simulink model "Ejercicio2"  (R2018b)
settings: Solver=FixedStepAuto  StartTime=0.0  StopTime=100.0  FixedStep=0.01  RelTol=1e-3
undefined symbols (not defined in the file or in its folder): DiscIntNeverNeededParam
libraries: simulink x1
settings Model: EnablePacing=on  PacingRate=10  Creator=Edu  LastModifiedBy=Edu

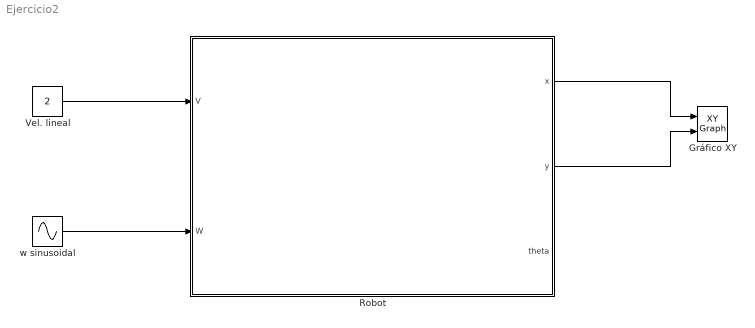
== system Ejercicio2 ==
  Gráfico XY : simulink/Sinks/XY Graph  xmin=-4  xmax=14  ymin=-4  ymax=14  st=-1
  Robot : Subsystem
  Vel. lineal : Constant  Value=2
  w sinusoidal : Sin  Amplitude=10  Frequency=10  SampleTime=0
  wires:
  Vel. lineal/1 -> Robot/1(V)
  Robot/1(x) -> Gráfico XY/1
  Robot/2(y) -> Gráfico XY/2
  w sinusoidal/1 -> Robot/2(W)

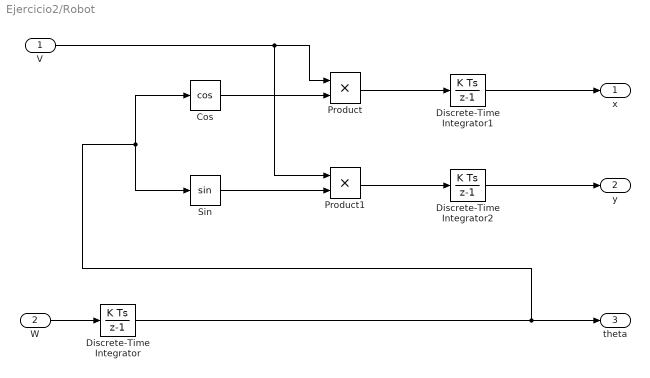
== system Ejercicio2/Robot ==
  V : Inport
  W : Inport  Port=2
  Cos : Trigonometry  Operator=cos
  Discrete-Time Integrator : DiscreteIntegrator  SampleTime=-1  ICPrevOutput=DiscIntNeverNeededParam  ICPrevScaledInput=DiscIntNeverNeededParam
  Discrete-Time Integrator1 : DiscreteIntegrator  InitialCondition=-4  SampleTime=-1  ICPrevOutput=DiscIntNeverNeededParam  ICPrevScaledInput=DiscIntNeverNeededParam
  Discrete-Time Integrator2 : DiscreteIntegrator  InitialCondition=-4  SampleTime=-1  ICPrevOutput=DiscIntNeverNeededParam  ICPrevScaledInput=DiscIntNeverNeededParam
  Product : Product
  Product1 : Product
  Sin : Trigonometry
  x : Outport
  y : Outport  Port=2
  theta : Outport  Port=3
  wires:
  Sin/1 -> Product1/2
  Product1/1 -> Discrete-Time Integrator2/1
  Product/1 -> Discrete-Time Integrator1/1
  Discrete-Time Integrator2/1 -> y/1
  V/1 -> Product1/1, Product/1
  Discrete-Time Integrator1/1 -> x/1
  Discrete-Time Integrator/1 -> Sin/1, Cos/1, theta/1
  W/1 -> Discrete-Time Integrator/1
  Cos/1 -> Product/2
